simulink model "Demo_veDYNA_cs"  (Simulink 7.6)
settings: Solver=ode1  SolverMode=SingleTasking  StartTime=0  StopTime=15  FixedStep=1/500  RelTol=1e-3
PreLoadFcn:
  | PreScanveDYNAPreLoadFcn(bdroot);
  | check_NUTS_defined;
  | 
  | assignin('base',['model_closed_' bdroot],false);
PostLoadFcn:
  | PreScanveDYNAPostLoadFcn(bdroot);
  | 
InitFcn:
  | vdy_SetExternalInputSource('ManLongCtrl',1,'Brake','other');
  | vdy_SetExternalInputSource('ManLongCtrl',1,'EngineTorque','other');
  | vdy_SetExternalInputSource('ManLatCtrl',1,'Steering','other');
  | 
  | PreScanveDYNAInitFcn(bdroot);
  | PreScanExperimentInitFcn(bdroot)
StopFcn:
  | PreScanExperimentStopFcn(bdroot)
undefined symbols (not defined in the file): at_period, CPT, DiscIntNeverNeededParam, vm_at_pulsewidth, vm_driver_dflt_gain, x_ini_VRML, y_ini_VRML, z_ini_VRML
libraries: dyna_cpt_lib x93, PreScanSimulinkLibrary x10, PreScanUsefulBlocks x4, simulink x4, anilib x3, dyna_lib x3, simulink_extras x2, dyna_manctrl_lib x2, dyna_road_lib x2, dyna_io_lib x1, dyna_demo_lib x1, dyna_usr_maneuver_states_lib x1
(part 6 of 8)

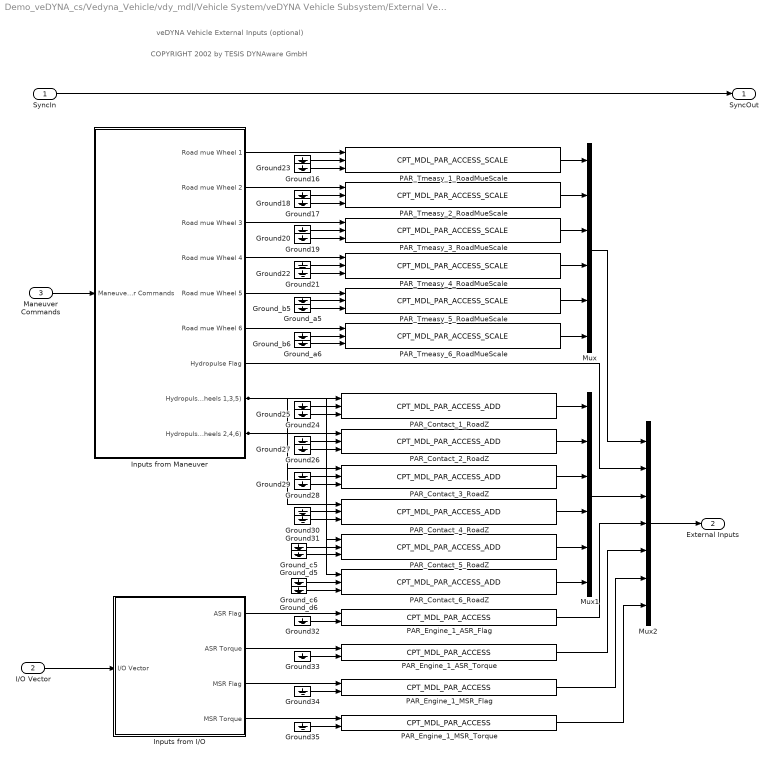
== system Demo_veDYNA_cs/Vedyna_Vehicle/vdy_mdl/Vehicle System/veDYNA Vehicle Subsystem/External Vehicle Inputs (from I/O) ==
  note: COPYRIGHT 2002 by TESIS DYNAware GmbH
  note: veDYNA Vehicle External Inputs (optional)
  SyncIn : Inport
  I/O Vector : Inport  Port=2
  Maneuver Commands : Inport  Port=3
  Ground{16..35} (20 alike) : Ground
  Ground_a5 : Ground
  Ground_a6 : Ground
  Ground_b5 : Ground
  Ground_b6 : Ground
  Ground_c5 : Ground
  Ground_c6 : Ground
  Ground_d5 : Ground
  Ground_d6 : Ground
  Inputs from I/O : Subsystem
  Inputs from Maneuver : Subsystem
  Mux : Mux  Inputs=6
  Mux1 : Mux  Inputs=6
  Mux2 : Mux  Inputs=7
  PAR_Contact_1_RoadZ : dyna_cpt_lib/CPT_MDL_PAR_ACCESS_ADD  Tag=vedynaCPT_MDL_PAR_ACCESS  component=Contact  system_inst=1  parameter=RoadZ
  PAR_Contact_2_RoadZ : dyna_cpt_lib/CPT_MDL_PAR_ACCESS_ADD  Tag=vedynaCPT_MDL_PAR_ACCESS  component=Contact  system_inst=2  parameter=RoadZ
  PAR_Contact_3_RoadZ : dyna_cpt_lib/CPT_MDL_PAR_ACCESS_ADD  Tag=vedynaCPT_MDL_PAR_ACCESS  component=Contact  system_inst=3  parameter=RoadZ
  PAR_Contact_4_RoadZ : dyna_cpt_lib/CPT_MDL_PAR_ACCESS_ADD  Tag=vedynaCPT_MDL_PAR_ACCESS  component=Contact  system_inst=4  parameter=RoadZ
  PAR_Contact_5_RoadZ : dyna_cpt_lib/CPT_MDL_PAR_ACCESS_ADD  Tag=vedynaCPT_MDL_PAR_ACCESS  component=Contact  system_inst=5  parameter=RoadZ
  PAR_Contact_6_RoadZ : dyna_cpt_lib/CPT_MDL_PAR_ACCESS_ADD  Tag=vedynaCPT_MDL_PAR_ACCESS  component=Contact  system_inst=6  parameter=RoadZ
  PAR_Engine_1_ASR_Flag : dyna_cpt_lib/CPT_MDL_PAR_ACCESS  Tag=vedynaCPT_MDL_PAR_ACCESS  component=Engine  system_inst=1  parameter=ASR_Flag
  PAR_Engine_1_ASR_Torque : dyna_cpt_lib/CPT_MDL_PAR_ACCESS  Tag=vedynaCPT_MDL_PAR_ACCESS  component=Engine  system_inst=1  parameter=ASR_Torque
  PAR_Engine_1_MSR_Flag : dyna_cpt_lib/CPT_MDL_PAR_ACCESS  Tag=vedynaCPT_MDL_PAR_ACCESS  component=Engine  system_inst=1  parameter=MSR_Flag
  PAR_Engine_1_MSR_Torque : dyna_cpt_lib/CPT_MDL_PAR_ACCESS  Tag=vedynaCPT_MDL_PAR_ACCESS  component=Engine  system_inst=1  parameter=MSR_Torque
  PAR_Tmeasy_1_RoadMueScale : dyna_cpt_lib/CPT_MDL_PAR_ACCESS_SCALE  Tag=vedynaCPT_MDL_PAR_ACCESS  component=Tmeasy  system_inst=1  parameter=RoadMueScale
  PAR_Tmeasy_2_RoadMueScale : dyna_cpt_lib/CPT_MDL_PAR_ACCESS_SCALE  Tag=vedynaCPT_MDL_PAR_ACCESS  component=Tmeasy  system_inst=2  parameter=RoadMueScale
  PAR_Tmeasy_3_RoadMueScale : dyna_cpt_lib/CPT_MDL_PAR_ACCESS_SCALE  Tag=vedynaCPT_MDL_PAR_ACCESS  component=Tmeasy  system_inst=3  parameter=RoadMueScale
  PAR_Tmeasy_4_RoadMueScale : dyna_cpt_lib/CPT_MDL_PAR_ACCESS_SCALE  Tag=vedynaCPT_MDL_PAR_ACCESS  component=Tmeasy  system_inst=4  parameter=RoadMueScale
  PAR_Tmeasy_5_RoadMueScale : dyna_cpt_lib/CPT_MDL_PAR_ACCESS_SCALE  Tag=vedynaCPT_MDL_PAR_ACCESS  component=Tmeasy  system_inst=5  parameter=RoadMueScale
  PAR_Tmeasy_6_RoadMueScale : dyna_cpt_lib/CPT_MDL_PAR_ACCESS_SCALE  Tag=vedynaCPT_MDL_PAR_ACCESS  component=Tmeasy  system_inst=6  parameter=RoadMueScale
  SyncOut : Outport
  External Inputs : Outport  Port=2
  wires:
  PAR_Contact_6_RoadZ/1 -> Mux1/6
  Ground_d6/1 -> PAR_Contact_6_RoadZ/3
  Ground_c6/1 -> PAR_Contact_6_RoadZ/2
  PAR_Contact_5_RoadZ/1 -> Mux1/5
  Ground_d5/1 -> PAR_Contact_5_RoadZ/3
  Ground_c5/1 -> PAR_Contact_5_RoadZ/2
  Inputs from Maneuver/9(Hydropulse Right (Wheels 2,4,6)) -> PAR_Contact_6_RoadZ/1, PAR_Contact_4_RoadZ/1, PAR_Contact_2_RoadZ/1
  Inputs from Maneuver/8(Hydropulse Left (Wheels 1,3,5)) -> PAR_Contact_5_RoadZ/1, PAR_Contact_3_RoadZ/1, PAR_Contact_1_RoadZ/1
  PAR_Tmeasy_6_RoadMueScale/1 -> Mux/6
  Inputs from Maneuver/6(Road mue Wheel 6) -> PAR_Tmeasy_6_RoadMueScale/1
  Ground_b6/1 -> PAR_Tmeasy_6_RoadMueScale/3
  Ground_a6/1 -> PAR_Tmeasy_6_RoadMueScale/2
  PAR_Tmeasy_5_RoadMueScale/1 -> Mux/5
  Inputs from Maneuver/5(Road mue Wheel 5) -> PAR_Tmeasy_5_RoadMueScale/1
  Ground_b5/1 -> PAR_Tmeasy_5_RoadMueScale/3
  Ground_a5/1 -> PAR_Tmeasy_5_RoadMueScale/2
  Ground16/1 -> PAR_Tmeasy_1_RoadMueScale/2
  Ground17/1 -> PAR_Tmeasy_2_RoadMueScale/2
  Ground18/1 -> PAR_Tmeasy_2_RoadMueScale/3
  Ground19/1 -> PAR_Tmeasy_3_RoadMueScale/2
  Ground20/1 -> PAR_Tmeasy_3_RoadMueScale/3
  Ground21/1 -> PAR_Tmeasy_4_RoadMueScale/2
  Ground22/1 -> PAR_Tmeasy_4_RoadMueScale/3
  Ground23/1 -> PAR_Tmeasy_1_RoadMueScale/3
  Ground24/1 -> PAR_Contact_1_RoadZ/2
  Ground25/1 -> PAR_Contact_1_RoadZ/3
  Ground26/1 -> PAR_Contact_2_RoadZ/2
  Ground27/1 -> PAR_Contact_2_RoadZ/3
  Ground28/1 -> PAR_Contact_3_RoadZ/2
  Ground29/1 -> PAR_Contact_3_RoadZ/3
  Ground30/1 -> PAR_Contact_4_RoadZ/2
  Ground31/1 -> PAR_Contact_4_RoadZ/3
  PAR_Tmeasy_1_RoadMueScale/1 -> Mux/1
  PAR_Tmeasy_2_RoadMueScale/1 -> Mux/2
  PAR_Contact_1_RoadZ/1 -> Mux1/1
  PAR_Contact_2_RoadZ/1 -> Mux1/2
  Inputs from Maneuver/1(Road mue Wheel 1) -> PAR_Tmeasy_1_RoadMueScale/1
  Inputs from Maneuver/2(Road mue Wheel 2) -> PAR_Tmeasy_2_RoadMueScale/1
  Inputs from Maneuver/3(Road mue Wheel 3) -> PAR_Tmeasy_3_RoadMueScale/1
  Inputs from Maneuver/4(Road mue Wheel 4) -> PAR_Tmeasy_4_RoadMueScale/1
  Maneuver Commands/1 -> Inputs from Maneuver/1(Maneuver Commands)
  SyncIn/1 -> SyncOut/1
  Ground32/1 -> PAR_Engine_1_ASR_Flag/2
  Ground33/1 -> PAR_Engine_1_ASR_Torque/2
  Ground34/1 -> PAR_Engine_1_MSR_Flag/2
  Ground35/1 -> PAR_Engine_1_MSR_Torque/2
  I/O Vector/1 -> Inputs from I/O/1(I/O Vector)
  Inputs from I/O/1(ASR Flag) -> PAR_Engine_1_ASR_Flag/1
  Inputs from I/O/2(ASR Torque) -> PAR_Engine_1_ASR_Torque/1
  Inputs from I/O/3(MSR Flag) -> PAR_Engine_1_MSR_Flag/1
  Inputs from I/O/4(MSR Torque) -> PAR_Engine_1_MSR_Torque/1
  PAR_Tmeasy_3_RoadMueScale/1 -> Mux/3
  PAR_Tmeasy_4_RoadMueScale/1 -> Mux/4
  PAR_Contact_3_RoadZ/1 -> Mux1/3
  PAR_Contact_4_RoadZ/1 -> Mux1/4
  Mux/1 -> Mux2/1
  Mux2/1 -> External Inputs/1
  Inputs from Maneuver/7(Hydropulse Flag) -> Mux2/2
  Mux1/1 -> Mux2/3
  PAR_Engine_1_ASR_Flag/1 -> Mux2/4
  PAR_Engine_1_ASR_Torque/1 -> Mux2/5
  PAR_Engine_1_MSR_Flag/1 -> Mux2/6
  PAR_Engine_1_MSR_Torque/1 -> Mux2/7

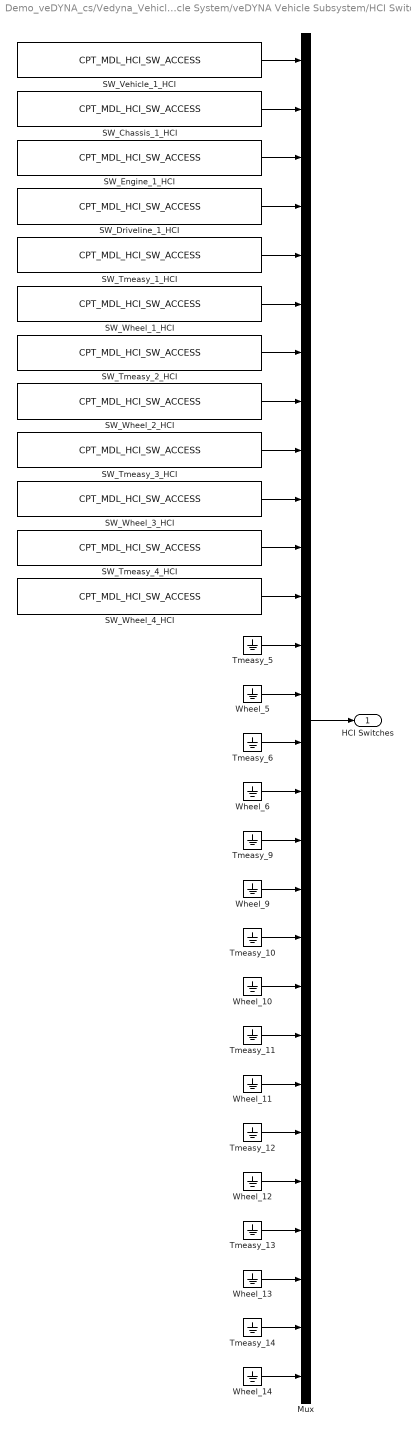
== system Demo_veDYNA_cs/Vedyna_Vehicle/vdy_mdl/Vehicle System/veDYNA Vehicle Subsystem/HCI Switches ==
  Mux : Mux  Inputs=28
  SW_Chassis_1_HCI : dyna_cpt_lib/CPT_MDL_HCI_SW_ACCESS  Tag=vedynaCPT_MDL_HCI_SW_ACCESS  component=Chassis  system_inst=1  parameter=HCI
  SW_Driveline_1_HCI : dyna_cpt_lib/CPT_MDL_HCI_SW_ACCESS  Tag=vedynaCPT_MDL_HCI_SW_ACCESS  component=Driveline  system_inst=1  parameter=HCI
  SW_Engine_1_HCI : dyna_cpt_lib/CPT_MDL_HCI_SW_ACCESS  Tag=vedynaCPT_MDL_HCI_SW_ACCESS  component=Engine  system_inst=1  parameter=HCI
  SW_Tmeasy_1_HCI : dyna_cpt_lib/CPT_MDL_HCI_SW_ACCESS  Tag=vedynaCPT_MDL_HCI_SW_ACCESS  component=Tmeasy  system_inst=1  parameter=HCI
  SW_Tmeasy_2_HCI : dyna_cpt_lib/CPT_MDL_HCI_SW_ACCESS  Tag=vedynaCPT_MDL_HCI_SW_ACCESS  component=Tmeasy  system_inst=2  parameter=HCI
  SW_Tmeasy_3_HCI : dyna_cpt_lib/CPT_MDL_HCI_SW_ACCESS  Tag=vedynaCPT_MDL_HCI_SW_ACCESS  component=Tmeasy  system_inst=3  parameter=HCI
  SW_Tmeasy_4_HCI : dyna_cpt_lib/CPT_MDL_HCI_SW_ACCESS  Tag=vedynaCPT_MDL_HCI_SW_ACCESS  component=Tmeasy  system_inst=4  parameter=HCI
  SW_Vehicle_1_HCI : dyna_cpt_lib/CPT_MDL_HCI_SW_ACCESS  Tag=vedynaCPT_MDL_HCI_SW_ACCESS  component=Vehicle  system_inst=1  parameter=HCI
  SW_Wheel_1_HCI : dyna_cpt_lib/CPT_MDL_HCI_SW_ACCESS  Tag=vedynaCPT_MDL_HCI_SW_ACCESS  component=Wheel  system_inst=1  parameter=HCI
  SW_Wheel_2_HCI : dyna_cpt_lib/CPT_MDL_HCI_SW_ACCESS  Tag=vedynaCPT_MDL_HCI_SW_ACCESS  component=Wheel  system_inst=2  parameter=HCI
  SW_Wheel_3_HCI : dyna_cpt_lib/CPT_MDL_HCI_SW_ACCESS  Tag=vedynaCPT_MDL_HCI_SW_ACCESS  component=Wheel  system_inst=3  parameter=HCI
  SW_Wheel_4_HCI : dyna_cpt_lib/CPT_MDL_HCI_SW_ACCESS  Tag=vedynaCPT_MDL_HCI_SW_ACCESS  component=Wheel  system_inst=4  parameter=HCI
  Tmeasy_{5..6,9..14} (8 alike) : Ground
  Wheel_{5..6,9..14} (8 alike) : Ground
  HCI Switches : Outport
  wires:
  Tmeasy_14/1 -> Mux/27
  Tmeasy_13/1 -> Mux/25
  Wheel_14/1 -> Mux/28
  Wheel_13/1 -> Mux/26
  Wheel_12/1 -> Mux/24
  Tmeasy_12/1 -> Mux/23
  Wheel_11/1 -> Mux/22
  Tmeasy_11/1 -> Mux/21
  Wheel_10/1 -> Mux/20
  Tmeasy_10/1 -> Mux/19
  Wheel_9/1 -> Mux/18
  Tmeasy_9/1 -> Mux/17
  Wheel_6/1 -> Mux/16
  Tmeasy_6/1 -> Mux/15
  Wheel_5/1 -> Mux/14
  Tmeasy_5/1 -> Mux/13
  SW_Wheel_4_HCI/1 -> Mux/12
  SW_Tmeasy_4_HCI/1 -> Mux/11
  SW_Wheel_3_HCI/1 -> Mux/10
  SW_Tmeasy_3_HCI/1 -> Mux/9
  SW_Wheel_2_HCI/1 -> Mux/8
  SW_Tmeasy_2_HCI/1 -> Mux/7
  SW_Wheel_1_HCI/1 -> Mux/6
  SW_Tmeasy_1_HCI/1 -> Mux/5
  SW_Driveline_1_HCI/1 -> Mux/4
  SW_Engine_1_HCI/1 -> Mux/3
  SW_Chassis_1_HCI/1 -> Mux/2
  SW_Vehicle_1_HCI/1 -> Mux/1
  Mux/1 -> HCI Switches/1

== system Demo_veDYNA_cs/Vedyna_Vehicle/vdy_mdl/Vehicle System/veDYNA Vehicle Subsystem/Maneuver Commands Splitter ==
  note: veDYNA Maneuver Command Splitter
  note: COPYRIGHT 2002 by TESIS DYNAware GmbH
  SyncIn : Inport
  Maneuver Commands : Inport  Port=2
  Demux : Demux  Outputs=[1,8,9]
  SyncOut : Outport
  Maneuver Commands to External Inputs : Outport  Port=2
  Maneuver Commands to Brake System : Outport  Port=3
  Maneuver Commands to Vehicle : Outport  Port=4
  wires:
  SyncIn/1 -> SyncOut/1
  Maneuver Commands/1 -> Demux/1
  Demux/3 -> Maneuver Commands to External Inputs/1
  Demux/1 -> Maneuver Commands to Brake System/1
  Demux/2 -> Maneuver Commands to Vehicle/1

== system Demo_veDYNA_cs/Vedyna_Vehicle/vdy_mdl/Vehicle System/veDYNA Vehicle Subsystem/Vehicle Outputs to I/O ==
  note: COPYRIGHT 2002 by TESIS DYNAware GmbH
  note: veDYNA Vehicle Interface to I/O (optional)
  SyncIn : Inport
  Read From WorkSpace : dyna_lib/Read From WorkSpace  comp=Wheel|Wheel|Wheel|Wheel|Wheel|Wheel|Wheel|Wheel  inst=0|1|2|3|4|5|6|7  group=wheelstate_v|wheelstate_v|wheelstate_v|wheelstate_v|wheelstate_v|wheelstate_v|wheelstate_v|wheelstate_v  var=or|or|or|or|or|or|or|or
  Output to IO : Outport
  SyncOut : Outport  Port=2
  wires:
  SyncIn/1 -> SyncOut/1
  Read From WorkSpace/1 -> Output to IO/1

== system Demo_veDYNA_cs/BMW_X5_1/Trajectories/Traj2State1/Traj2State2/Traj2MuxState_Ext/demux ==
  traj : Inport
  Demux : Demux  Outputs=18
  x : Outport
  y : Outport  Port=2
  z : Outport  Port=3
  velx : Outport  Port=4
  vely : Outport  Port=5
  velz : Outport  Port=6
  R : Outport  Port=7
  P : Outport  Port=8
  Y : Outport  Port=9
  velR : Outport  Port=10
  velP : Outport  Port=11
  velY : Outport  Port=12
  accx : Outport  Port=13
  accy : Outport  Port=14
  accz : Outport  Port=15
  accR : Outport  Port=16
  accP : Outport  Port=17
  accY : Outport  Port=18
  wires:
  Demux/18 -> accY/1
  Demux/17 -> accP/1
  Demux/16 -> accR/1
  Demux/15 -> accz/1
  Demux/14 -> accy/1
  Demux/13 -> accx/1
  Demux/12 -> velY/1
  Demux/11 -> velP/1
  Demux/10 -> velR/1
  Demux/9 -> velz/1
  Demux/8 -> vely/1
  Demux/7 -> velx/1
  Demux/6 -> Y/1
  Demux/5 -> P/1
  traj/1 -> Demux/1
  Demux/4 -> R/1
  Demux/3 -> z/1
  Demux/2 -> y/1
  Demux/1 -> x/1

== system Demo_veDYNA_cs/Nissan_Cabstar_1/Trajectories/Traj2State1/Traj2State2/Traj2MuxState_Ext/demux ==
  traj : Inport
  Demux : Demux  Outputs=18
  x : Outport
  y : Outport  Port=2
  z : Outport  Port=3
  velx : Outport  Port=4
  vely : Outport  Port=5
  velz : Outport  Port=6
  R : Outport  Port=7
  P : Outport  Port=8
  Y : Outport  Port=9
  velR : Outport  Port=10
  velP : Outport  Port=11
  velY : Outport  Port=12
  accx : Outport  Port=13
  accy : Outport  Port=14
  accz : Outport  Port=15
  accR : Outport  Port=16
  accP : Outport  Port=17
  accY : Outport  Port=18
  wires:
  Demux/18 -> accY/1
  Demux/17 -> accP/1
  Demux/16 -> accR/1
  Demux/15 -> accz/1
  Demux/14 -> accy/1
  Demux/13 -> accx/1
  Demux/12 -> velY/1
  Demux/11 -> velP/1
  Demux/10 -> velR/1
  Demux/9 -> velz/1
  Demux/8 -> vely/1
  Demux/7 -> velx/1
  Demux/6 -> Y/1
  Demux/5 -> P/1
  traj/1 -> Demux/1
  Demux/4 -> R/1
  Demux/3 -> z/1
  Demux/2 -> y/1
  Demux/1 -> x/1

== system Demo_veDYNA_cs/Vedyna_Vehicle/CPT_MDL/MDL_PAR/BrkHyd/System Instance 1/pbrmaster [N/m**2] ==
  Table : Lookup  InputValues=CPT.MDL_PAR.BrkHyd{1}.pbrmaster.Table.x  Table=CPT.MDL_PAR.BrkHyd{1}.pbrmaster.Table.v  SaturateOnIntegerOverflow=on
  Terminator : Terminator
  Terminator1 : Terminator
  Value : Constant  Value=CPT.MDL_PAR.BrkHyd{1}.pbrmaster.Value.v
  tag scope: BrkHyd_1_pbrmaster_TBL=global, BrkHyd_1_pbrmaster_VAL=global
  wires:
  [vdy_Simctrl_tsim] -> Table/1
  Value/1 -> [BrkHyd_1_pbrmaster_VAL]
  [BrkHyd_1_pbrmaster_VAL] -> Terminator/1
  [BrkHyd_1_pbrmaster_TBL] -> Terminator1/1
  Table/1 -> [BrkHyd_1_pbrmaster_TBL]

== system Demo_veDYNA_cs/Vedyna_Vehicle/CPT_MDL/MDL_PAR/ClutchCtrl/System Instance 1/Clutch [%] ==
  Table : Lookup  InputValues=CPT.MDL_PAR.ClutchCtrl{1}.Clutch.Table.x  Table=CPT.MDL_PAR.ClutchCtrl{1}.Clutch.Table.v  SaturateOnIntegerOverflow=on
  Terminator : Terminator
  Terminator1 : Terminator
  Value : Constant  Value=CPT.MDL_PAR.ClutchCtrl{1}.Clutch.Value.v
  tag scope: ClutchCtrl_1_Clutch_TBL=global, ClutchCtrl_1_Clutch_VAL=global
  wires:
  [vdy_Simctrl_tsim] -> Table/1
  Value/1 -> [ClutchCtrl_1_Clutch_VAL]
  [ClutchCtrl_1_Clutch_VAL] -> Terminator/1
  [ClutchCtrl_1_Clutch_TBL] -> Terminator1/1
  Table/1 -> [ClutchCtrl_1_Clutch_TBL]

== system Demo_veDYNA_cs/Vedyna_Vehicle/CPT_MDL/MDL_PAR/Contact/System Instance 1/RoadZ [m] ==
  Table : Lookup  InputValues=CPT.MDL_PAR.Contact{1}.RoadZ.Table.x  Table=CPT.MDL_PAR.Contact{1}.RoadZ.Table.v  SaturateOnIntegerOverflow=on
  Terminator : Terminator
  Terminator1 : Terminator
  Value : Constant  Value=CPT.MDL_PAR.Contact{1}.RoadZ.Value.v
  tag scope: Contact_1_RoadZ_TBL=global, Contact_1_RoadZ_VAL=global
  wires:
  [vdy_Simctrl_tsim] -> Table/1
  Value/1 -> [Contact_1_RoadZ_VAL]
  [Contact_1_RoadZ_VAL] -> Terminator/1
  [Contact_1_RoadZ_TBL] -> Terminator1/1
  Table/1 -> [Contact_1_RoadZ_TBL]

== system Demo_veDYNA_cs/Vedyna_Vehicle/CPT_MDL/MDL_PAR/Contact/System Instance 2/RoadZ [m] ==
  Table : Lookup  InputValues=CPT.MDL_PAR.Contact{2}.RoadZ.Table.x  Table=CPT.MDL_PAR.Contact{2}.RoadZ.Table.v  SaturateOnIntegerOverflow=on
  Terminator : Terminator
  Terminator1 : Terminator
  Value : Constant  Value=CPT.MDL_PAR.Contact{2}.RoadZ.Value.v
  tag scope: Contact_2_RoadZ_TBL=global, Contact_2_RoadZ_VAL=global
  wires:
  [vdy_Simctrl_tsim] -> Table/1
  Value/1 -> [Contact_2_RoadZ_VAL]
  [Contact_2_RoadZ_VAL] -> Terminator/1
  [Contact_2_RoadZ_TBL] -> Terminator1/1
  Table/1 -> [Contact_2_RoadZ_TBL]

== system Demo_veDYNA_cs/Vedyna_Vehicle/CPT_MDL/MDL_PAR/Contact/System Instance 3/RoadZ [m] ==
  Table : Lookup  InputValues=CPT.MDL_PAR.Contact{3}.RoadZ.Table.x  Table=CPT.MDL_PAR.Contact{3}.RoadZ.Table.v  SaturateOnIntegerOverflow=on
  Terminator : Terminator
  Terminator1 : Terminator
  Value : Constant  Value=CPT.MDL_PAR.Contact{3}.RoadZ.Value.v
  tag scope: Contact_3_RoadZ_TBL=global, Contact_3_RoadZ_VAL=global
  wires:
  [vdy_Simctrl_tsim] -> Table/1
  Value/1 -> [Contact_3_RoadZ_VAL]
  [Contact_3_RoadZ_VAL] -> Terminator/1
  [Contact_3_RoadZ_TBL] -> Terminator1/1
  Table/1 -> [Contact_3_RoadZ_TBL]

== system Demo_veDYNA_cs/Vedyna_Vehicle/CPT_MDL/MDL_PAR/Contact/System Instance 4/RoadZ [m] ==
  Table : Lookup  InputValues=CPT.MDL_PAR.Contact{4}.RoadZ.Table.x  Table=CPT.MDL_PAR.Contact{4}.RoadZ.Table.v  SaturateOnIntegerOverflow=on
  Terminator : Terminator
  Terminator1 : Terminator
  Value : Constant  Value=CPT.MDL_PAR.Contact{4}.RoadZ.Value.v
  tag scope: Contact_4_RoadZ_TBL=global, Contact_4_RoadZ_VAL=global
  wires:
  [vdy_Simctrl_tsim] -> Table/1
  Value/1 -> [Contact_4_RoadZ_VAL]
  [Contact_4_RoadZ_VAL] -> Terminator/1
  [Contact_4_RoadZ_TBL] -> Terminator1/1
  Table/1 -> [Contact_4_RoadZ_TBL]

== system Demo_veDYNA_cs/Vedyna_Vehicle/CPT_MDL/MDL_PAR/Contact/System Instance 5/RoadZ [m] ==
  Table : Lookup  InputValues=CPT.MDL_PAR.Contact{5}.RoadZ.Table.x  Table=CPT.MDL_PAR.Contact{5}.RoadZ.Table.v  SaturateOnIntegerOverflow=on
  Terminator : Terminator
  Terminator1 : Terminator
  Value : Constant  Value=CPT.MDL_PAR.Contact{5}.RoadZ.Value.v
  tag scope: Contact_5_RoadZ_TBL=global, Contact_5_RoadZ_VAL=global
  wires:
  [vdy_Simctrl_tsim] -> Table/1
  Value/1 -> [Contact_5_RoadZ_VAL]
  [Contact_5_RoadZ_VAL] -> Terminator/1
  [Contact_5_RoadZ_TBL] -> Terminator1/1
  Table/1 -> [Contact_5_RoadZ_TBL]

== system Demo_veDYNA_cs/Vedyna_Vehicle/CPT_MDL/MDL_PAR/Contact/System Instance 6/RoadZ [m] ==
  Table : Lookup  InputValues=CPT.MDL_PAR.Contact{6}.RoadZ.Table.x  Table=CPT.MDL_PAR.Contact{6}.RoadZ.Table.v  SaturateOnIntegerOverflow=on
  Terminator : Terminator
  Terminator1 : Terminator
  Value : Constant  Value=CPT.MDL_PAR.Contact{6}.RoadZ.Value.v
  tag scope: Contact_6_RoadZ_TBL=global, Contact_6_RoadZ_VAL=global
  wires:
  [vdy_Simctrl_tsim] -> Table/1
  Value/1 -> [Contact_6_RoadZ_VAL]
  [Contact_6_RoadZ_VAL] -> Terminator/1
  [Contact_6_RoadZ_TBL] -> Terminator1/1
  Table/1 -> [Contact_6_RoadZ_TBL]

== system Demo_veDYNA_cs/Vedyna_Vehicle/CPT_MDL/MDL_PAR/Contact/System Instance 7/RoadZ [m] ==
  Table : Lookup  InputValues=CPT.MDL_PAR.Contact{7}.RoadZ.Table.x  Table=CPT.MDL_PAR.Contact{7}.RoadZ.Table.v  SaturateOnIntegerOverflow=on
  Terminator : Terminator
  Terminator1 : Terminator
  Value : Constant  Value=CPT.MDL_PAR.Contact{7}.RoadZ.Value.v
  tag scope: Contact_7_RoadZ_TBL=global, Contact_7_RoadZ_VAL=global
  wires:
  [vdy_Simctrl_tsim] -> Table/1
  Value/1 -> [Contact_7_RoadZ_VAL]
  [Contact_7_RoadZ_VAL] -> Terminator/1
  [Contact_7_RoadZ_TBL] -> Terminator1/1
  Table/1 -> [Contact_7_RoadZ_TBL]

== system Demo_veDYNA_cs/Vedyna_Vehicle/CPT_MDL/MDL_PAR/Contact/System Instance 8/RoadZ [m] ==
  Table : Lookup  InputValues=CPT.MDL_PAR.Contact{8}.RoadZ.Table.x  Table=CPT.MDL_PAR.Contact{8}.RoadZ.Table.v  SaturateOnIntegerOverflow=on
  Terminator : Terminator
  Terminator1 : Terminator
  Value : Constant  Value=CPT.MDL_PAR.Contact{8}.RoadZ.Value.v
  tag scope: Contact_8_RoadZ_TBL=global, Contact_8_RoadZ_VAL=global
  wires:
  [vdy_Simctrl_tsim] -> Table/1
  Value/1 -> [Contact_8_RoadZ_VAL]
  [Contact_8_RoadZ_VAL] -> Terminator/1
  [Contact_8_RoadZ_TBL] -> Terminator1/1
  Table/1 -> [Contact_8_RoadZ_TBL]

== system Demo_veDYNA_cs/Vedyna_Vehicle/CPT_MDL/MDL_PAR/Driver/System Instance 1/acc_comp_scale [-] ==
  Table : Lookup  InputValues=CPT.MDL_PAR.Driver{1}.acc_comp_scale.Table.x  Table=CPT.MDL_PAR.Driver{1}.acc_comp_scale.Table.v  SaturateOnIntegerOverflow=on
  Terminator : Terminator
  Terminator1 : Terminator
  Value : Constant  Value=CPT.MDL_PAR.Driver{1}.acc_comp_scale.Value.v
  tag scope: Driver_1_acc_comp_scale_TBL=global, Driver_1_acc_comp_scale_VAL=global
  wires:
  [vdy_Simctrl_tsim] -> Table/1
  Value/1 -> [Driver_1_acc_comp_scale_VAL]
  [Driver_1_acc_comp_scale_VAL] -> Terminator/1
  [Driver_1_acc_comp_scale_TBL] -> Terminator1/1
  Table/1 -> [Driver_1_acc_comp_scale_TBL]

== system Demo_veDYNA_cs/Vedyna_Vehicle/CPT_MDL/MDL_PAR/Driver/System Instance 1/adj_acc_gain [-] ==
  Table : Lookup  InputValues=CPT.MDL_PAR.Driver{1}.adj_acc_gain.Table.x  Table=CPT.MDL_PAR.Driver{1}.adj_acc_gain.Table.v  SaturateOnIntegerOverflow=on
  Terminator : Terminator
  Terminator1 : Terminator
  Value : Constant  Value=CPT.MDL_PAR.Driver{1}.adj_acc_gain.Value.v
  tag scope: Driver_1_adj_acc_gain_TBL=global, Driver_1_adj_acc_gain_VAL=global
  wires:
  [vdy_Simctrl_tsim] -> Table/1
  Value/1 -> [Driver_1_adj_acc_gain_VAL]
  [Driver_1_adj_acc_gain_VAL] -> Terminator/1
  [Driver_1_adj_acc_gain_TBL] -> Terminator1/1
  Table/1 -> [Driver_1_adj_acc_gain_TBL]

== system Demo_veDYNA_cs/Vedyna_Vehicle/CPT_MDL/MDL_PAR/Driver/System Instance 1/adj_brake_gain [-] ==
  Table : Lookup  InputValues=CPT.MDL_PAR.Driver{1}.adj_brake_gain.Table.x  Table=CPT.MDL_PAR.Driver{1}.adj_brake_gain.Table.v  SaturateOnIntegerOverflow=on
  Terminator : Terminator
  Terminator1 : Terminator
  Value : Constant  Value=CPT.MDL_PAR.Driver{1}.adj_brake_gain.Value.v
  tag scope: Driver_1_adj_brake_gain_TBL=global, Driver_1_adj_brake_gain_VAL=global
  wires:
  [vdy_Simctrl_tsim] -> Table/1
  Value/1 -> [Driver_1_adj_brake_gain_VAL]
  [Driver_1_adj_brake_gain_VAL] -> Terminator/1
  [Driver_1_adj_brake_gain_TBL] -> Terminator1/1
  Table/1 -> [Driver_1_adj_brake_gain_TBL]

== system Demo_veDYNA_cs/Vedyna_Vehicle/CPT_MDL/MDL_PAR/Driver/System Instance 1/ax_min [m/s^2] ==
  Table : Lookup  InputValues=CPT.MDL_PAR.Driver{1}.ax_min.Table.x  Table=CPT.MDL_PAR.Driver{1}.ax_min.Table.v  SaturateOnIntegerOverflow=on
  Terminator : Terminator
  Terminator1 : Terminator
  Value : Constant  Value=CPT.MDL_PAR.Driver{1}.ax_min.Value.v
  tag scope: Driver_1_ax_min_TBL=global, Driver_1_ax_min_VAL=global
  wires:
  [vdy_Simctrl_tsim] -> Table/1
  Value/1 -> [Driver_1_ax_min_VAL]
  [Driver_1_ax_min_VAL] -> Terminator/1
  [Driver_1_ax_min_TBL] -> Terminator1/1
  Table/1 -> [Driver_1_ax_min_TBL]

== system Demo_veDYNA_cs/Vedyna_Vehicle/CPT_MDL/MDL_PAR/Driver/System Instance 1/ctrl_acc_smooth_t [s] ==
  Table : Lookup  InputValues=CPT.MDL_PAR.Driver{1}.ctrl_acc_smooth_t.Table.x  Table=CPT.MDL_PAR.Driver{1}.ctrl_acc_smooth_t.Table.v  SaturateOnIntegerOverflow=on
  Terminator : Terminator
  Terminator1 : Terminator
  Value : Constant  Value=CPT.MDL_PAR.Driver{1}.ctrl_acc_smooth_t.Value.v
  tag scope: Driver_1_ctrl_acc_smooth_t_TBL=global, Driver_1_ctrl_acc_smooth_t_VAL=global
  wires:
  [vdy_Simctrl_tsim] -> Table/1
  Value/1 -> [Driver_1_ctrl_acc_smooth_t_VAL]
  [Driver_1_ctrl_acc_smooth_t_VAL] -> Terminator/1
  [Driver_1_ctrl_acc_smooth_t_TBL] -> Terminator1/1
  Table/1 -> [Driver_1_ctrl_acc_smooth_t_TBL]

== system Demo_veDYNA_cs/Vedyna_Vehicle/CPT_MDL/MDL_PAR/Driver/System Instance 1/cu_comp_scale [-] ==
  Table : Lookup  InputValues=CPT.MDL_PAR.Driver{1}.cu_comp_scale.Table.x  Table=CPT.MDL_PAR.Driver{1}.cu_comp_scale.Table.v  SaturateOnIntegerOverflow=on
  Terminator : Terminator
  Terminator1 : Terminator
  Value : Constant  Value=CPT.MDL_PAR.Driver{1}.cu_comp_scale.Value.v
  tag scope: Driver_1_cu_comp_scale_TBL=global, Driver_1_cu_comp_scale_VAL=global
  wires:
  [vdy_Simctrl_tsim] -> Table/1
  Value/1 -> [Driver_1_cu_comp_scale_VAL]
  [Driver_1_cu_comp_scale_VAL] -> Terminator/1
  [Driver_1_cu_comp_scale_TBL] -> Terminator1/1
  Table/1 -> [Driver_1_cu_comp_scale_TBL]

== system Demo_veDYNA_cs/Vedyna_Vehicle/CPT_MDL/MDL_PAR/Driver/System Instance 1/cu_path [1/m] ==
  Table : Lookup  InputValues=CPT.MDL_PAR.Driver{1}.cu_path.Table.x  Table=CPT.MDL_PAR.Driver{1}.cu_path.Table.v  SaturateOnIntegerOverflow=on
  Terminator : Terminator
  Terminator1 : Terminator
  Value : Constant  Value=CPT.MDL_PAR.Driver{1}.cu_path.Value.v
  tag scope: Driver_1_cu_path_TBL=global, Driver_1_cu_path_VAL=global
  wires:
  [vdy_Driver_s] -> Table/1
  Value/1 -> [Driver_1_cu_path_VAL]
  [Driver_1_cu_path_VAL] -> Terminator/1
  [Driver_1_cu_path_TBL] -> Terminator1/1
  Table/1 -> [Driver_1_cu_path_TBL]

== system Demo_veDYNA_cs/Vedyna_Vehicle/CPT_MDL/MDL_PAR/Driver/System Instance 1/front_stiff [N/rad] ==
  Table : Lookup  InputValues=CPT.MDL_PAR.Driver{1}.front_stiff.Table.x  Table=CPT.MDL_PAR.Driver{1}.front_stiff.Table.v  SaturateOnIntegerOverflow=on
  Terminator : Terminator
  Terminator1 : Terminator
  Value : Constant  Value=CPT.MDL_PAR.Driver{1}.front_stiff.Value.v
  tag scope: Driver_1_front_stiff_TBL=global, Driver_1_front_stiff_VAL=global
  wires:
  [vdy_Simctrl_tsim] -> Table/1
  Value/1 -> [Driver_1_front_stiff_VAL]
  [Driver_1_front_stiff_VAL] -> Terminator/1
  [Driver_1_front_stiff_TBL] -> Terminator1/1
  Table/1 -> [Driver_1_front_stiff_TBL]

== system Demo_veDYNA_cs/Vedyna_Vehicle/CPT_MDL/MDL_PAR/Driver/System Instance 1/front_stiff_sw [-] ==
  Table : Lookup  InputValues=CPT.MDL_PAR.Driver{1}.front_stiff_sw.Table.x  Table=CPT.MDL_PAR.Driver{1}.front_stiff_sw.Table.v  SaturateOnIntegerOverflow=on
  Terminator : Terminator
  Terminator1 : Terminator
  Value : Constant  Value=CPT.MDL_PAR.Driver{1}.front_stiff_sw.Value.v
  tag scope: Driver_1_front_stiff_sw_TBL=global, Driver_1_front_stiff_sw_VAL=global
  wires:
  [vdy_Simctrl_tsim] -> Table/1
  Value/1 -> [Driver_1_front_stiff_sw_VAL]
  [Driver_1_front_stiff_sw_VAL] -> Terminator/1
  [Driver_1_front_stiff_sw_TBL] -> Terminator1/1
  Table/1 -> [Driver_1_front_stiff_sw_TBL]

== system Demo_veDYNA_cs/Vedyna_Vehicle/CPT_MDL/MDL_PAR/Driver/System Instance 1/gain_lat [-] ==
  Table : Lookup  InputValues=CPT.MDL_PAR.Driver{1}.gain_lat.Table.x  Table=CPT.MDL_PAR.Driver{1}.gain_lat.Table.v  SaturateOnIntegerOverflow=on
  Terminator : Terminator
  Terminator1 : Terminator
  Value : Constant  Value=CPT.MDL_PAR.Driver{1}.gain_lat.Value.v
  tag scope: Driver_1_gain_lat_TBL=global, Driver_1_gain_lat_VAL=global
  wires:
  [vdy_Simctrl_tsim] -> Table/1
  Value/1 -> [Driver_1_gain_lat_VAL]
  [Driver_1_gain_lat_VAL] -> Terminator/1
  [Driver_1_gain_lat_TBL] -> Terminator1/1
  Table/1 -> [Driver_1_gain_lat_TBL]

== system Demo_veDYNA_cs/Vedyna_Vehicle/CPT_MDL/MDL_PAR/Driver/System Instance 1/gain_long [-] ==
  Table : Lookup  InputValues=CPT.MDL_PAR.Driver{1}.gain_long.Table.x  Table=CPT.MDL_PAR.Driver{1}.gain_long.Table.v  SaturateOnIntegerOverflow=on
  Terminator : Terminator
  Terminator1 : Terminator
  Value : Constant  Value=CPT.MDL_PAR.Driver{1}.gain_long.Value.v
  tag scope: Driver_1_gain_long_TBL=global, Driver_1_gain_long_VAL=global
  wires:
  [vdy_Simctrl_tsim] -> Table/1
  Value/1 -> [Driver_1_gain_long_VAL]
  [Driver_1_gain_long_VAL] -> Terminator/1
  [Driver_1_gain_long_TBL] -> Terminator1/1
  Table/1 -> [Driver_1_gain_long_TBL]

== system Demo_veDYNA_cs/Vedyna_Vehicle/CPT_MDL/MDL_PAR/Driver/System Instance 1/lat_for_r_scale [-] ==
  Table : Lookup  InputValues=CPT.MDL_PAR.Driver{1}.lat_for_r_scale.Table.x  Table=CPT.MDL_PAR.Driver{1}.lat_for_r_scale.Table.v  SaturateOnIntegerOverflow=on
  Terminator : Terminator
  Terminator1 : Terminator
  Value : Constant  Value=CPT.MDL_PAR.Driver{1}.lat_for_r_scale.Value.v
  tag scope: Driver_1_lat_for_r_scale_TBL=global, Driver_1_lat_for_r_scale_VAL=global
  wires:
  [vdy_Simctrl_tsim] -> Table/1
  Value/1 -> [Driver_1_lat_for_r_scale_VAL]
  [Driver_1_lat_for_r_scale_VAL] -> Terminator/1
  [Driver_1_lat_for_r_scale_TBL] -> Terminator1/1
  Table/1 -> [Driver_1_lat_for_r_scale_TBL]

== system Demo_veDYNA_cs/Vedyna_Vehicle/CPT_MDL/MDL_PAR/Driver/System Instance 1/lat_for_r_smooth_t [s] ==
  Table : Lookup  InputValues=CPT.MDL_PAR.Driver{1}.lat_for_r_smooth_t.Table.x  Table=CPT.MDL_PAR.Driver{1}.lat_for_r_smooth_t.Table.v  SaturateOnIntegerOverflow=on
  Terminator : Terminator
  Terminator1 : Terminator
  Value : Constant  Value=CPT.MDL_PAR.Driver{1}.lat_for_r_smooth_t.Value.v
  tag scope: Driver_1_lat_for_r_smooth_t_TBL=global, Driver_1_lat_for_r_smooth_t_VAL=global
  wires:
  [vdy_Simctrl_tsim] -> Table/1
  Value/1 -> [Driver_1_lat_for_r_smooth_t_VAL]
  [Driver_1_lat_for_r_smooth_t_VAL] -> Terminator/1
  [Driver_1_lat_for_r_smooth_t_TBL] -> Terminator1/1
  Table/1 -> [Driver_1_lat_for_r_smooth_t_TBL]

== system Demo_veDYNA_cs/Vedyna_Vehicle/CPT_MDL/MDL_PAR/Driver/System Instance 1/lat_for_r_sw [-] ==
  Table : Lookup  InputValues=CPT.MDL_PAR.Driver{1}.lat_for_r_sw.Table.x  Table=CPT.MDL_PAR.Driver{1}.lat_for_r_sw.Table.v  SaturateOnIntegerOverflow=on
  Terminator : Terminator
  Terminator1 : Terminator
  Value : Constant  Value=CPT.MDL_PAR.Driver{1}.lat_for_r_sw.Value.v
  tag scope: Driver_1_lat_for_r_sw_TBL=global, Driver_1_lat_for_r_sw_VAL=global
  wires:
  [vdy_Simctrl_tsim] -> Table/1
  Value/1 -> [Driver_1_lat_for_r_sw_VAL]
  [Driver_1_lat_for_r_sw_VAL] -> Terminator/1
  [Driver_1_lat_for_r_sw_TBL] -> Terminator1/1
  Table/1 -> [Driver_1_lat_for_r_sw_TBL]

== system Demo_veDYNA_cs/Vedyna_Vehicle/CPT_MDL/MDL_PAR/Driver/System Instance 1/path_v_scale [-] ==
  Table : Lookup  InputValues=CPT.MDL_PAR.Driver{1}.path_v_scale.Table.x  Table=CPT.MDL_PAR.Driver{1}.path_v_scale.Table.v  SaturateOnIntegerOverflow=on
  Terminator : Terminator
  Terminator1 : Terminator
  Value : Constant  Value=CPT.MDL_PAR.Driver{1}.path_v_scale.Value.v
  tag scope: Driver_1_path_v_scale_TBL=global, Driver_1_path_v_scale_VAL=global
  wires:
  [vdy_Simctrl_tsim] -> Table/1
  Value/1 -> [Driver_1_path_v_scale_VAL]
  [Driver_1_path_v_scale_VAL] -> Terminator/1
  [Driver_1_path_v_scale_TBL] -> Terminator1/1
  Table/1 -> [Driver_1_path_v_scale_TBL]

== system Demo_veDYNA_cs/Vedyna_Vehicle/CPT_MDL/MDL_PAR/Driver/System Instance 1/path_x_offset [m] ==
  Table : Lookup  InputValues=CPT.MDL_PAR.Driver{1}.path_x_offset.Table.x  Table=CPT.MDL_PAR.Driver{1}.path_x_offset.Table.v  SaturateOnIntegerOverflow=on
  Terminator : Terminator
  Terminator1 : Terminator
  Value : Constant  Value=CPT.MDL_PAR.Driver{1}.path_x_offset.Value.v
  tag scope: Driver_1_path_x_offset_TBL=global, Driver_1_path_x_offset_VAL=global
  wires:
  [vdy_Simctrl_tsim] -> Table/1
  Value/1 -> [Driver_1_path_x_offset_VAL]
  [Driver_1_path_x_offset_VAL] -> Terminator/1
  [Driver_1_path_x_offset_TBL] -> Terminator1/1
  Table/1 -> [Driver_1_path_x_offset_TBL]

== system Demo_veDYNA_cs/Vedyna_Vehicle/CPT_MDL/MDL_PAR/Driver/System Instance 1/psi_path [rad] ==
  Table : Lookup  InputValues=CPT.MDL_PAR.Driver{1}.psi_path.Table.x  Table=CPT.MDL_PAR.Driver{1}.psi_path.Table.v  SaturateOnIntegerOverflow=on
  Terminator : Terminator
  Terminator1 : Terminator
  Value : Constant  Value=CPT.MDL_PAR.Driver{1}.psi_path.Value.v
  tag scope: Driver_1_psi_path_TBL=global, Driver_1_psi_path_VAL=global
  wires:
  [vdy_Driver_s] -> Table/1
  Value/1 -> [Driver_1_psi_path_VAL]
  [Driver_1_psi_path_VAL] -> Terminator/1
  [Driver_1_psi_path_TBL] -> Terminator1/1
  Table/1 -> [Driver_1_psi_path_TBL]

== system Demo_veDYNA_cs/Vedyna_Vehicle/CPT_MDL/MDL_PAR/Driver/System Instance 1/q_path [m] ==
  Table : Lookup  InputValues=CPT.MDL_PAR.Driver{1}.q_path.Table.x  Table=CPT.MDL_PAR.Driver{1}.q_path.Table.v  SaturateOnIntegerOverflow=on
  Terminator : Terminator
  Terminator1 : Terminator
  Value : Constant  Value=CPT.MDL_PAR.Driver{1}.q_path.Value.v
  tag scope: Driver_1_q_path_TBL=global, Driver_1_q_path_VAL=global
  wires:
  [vdy_Driver_s] -> Table/1
  Value/1 -> [Driver_1_q_path_VAL]
  [Driver_1_q_path_VAL] -> Terminator/1
  [Driver_1_q_path_TBL] -> Terminator1/1
  Table/1 -> [Driver_1_q_path_TBL]

== system Demo_veDYNA_cs/Vedyna_Vehicle/CPT_MDL/MDL_PAR/Driver/System Instance 1/rear_stiff [N/rad] ==
  Table : Lookup  InputValues=CPT.MDL_PAR.Driver{1}.rear_stiff.Table.x  Table=CPT.MDL_PAR.Driver{1}.rear_stiff.Table.v  SaturateOnIntegerOverflow=on
  Terminator : Terminator
  Terminator1 : Terminator
  Value : Constant  Value=CPT.MDL_PAR.Driver{1}.rear_stiff.Value.v
  tag scope: Driver_1_rear_stiff_TBL=global, Driver_1_rear_stiff_VAL=global
  wires:
  [vdy_Simctrl_tsim] -> Table/1
  Value/1 -> [Driver_1_rear_stiff_VAL]
  [Driver_1_rear_stiff_VAL] -> Terminator/1
  [Driver_1_rear_stiff_TBL] -> Terminator1/1
  Table/1 -> [Driver_1_rear_stiff_TBL]

== system Demo_veDYNA_cs/Vedyna_Vehicle/CPT_MDL/MDL_PAR/Driver/System Instance 1/rear_stiff_sw [-] ==
  Table : Lookup  InputValues=CPT.MDL_PAR.Driver{1}.rear_stiff_sw.Table.x  Table=CPT.MDL_PAR.Driver{1}.rear_stiff_sw.Table.v  SaturateOnIntegerOverflow=on
  Terminator : Terminator
  Terminator1 : Terminator
  Value : Constant  Value=CPT.MDL_PAR.Driver{1}.rear_stiff_sw.Value.v
  tag scope: Driver_1_rear_stiff_sw_TBL=global, Driver_1_rear_stiff_sw_VAL=global
  wires:
  [vdy_Simctrl_tsim] -> Table/1
  Value/1 -> [Driver_1_rear_stiff_sw_VAL]
  [Driver_1_rear_stiff_sw_VAL] -> Terminator/1
  [Driver_1_rear_stiff_sw_TBL] -> Terminator1/1
  Table/1 -> [Driver_1_rear_stiff_sw_TBL]

== system Demo_veDYNA_cs/Vedyna_Vehicle/CPT_MDL/MDL_PAR/Driver/System Instance 1/steer_max [deg] ==
  Table : Lookup  InputValues=CPT.MDL_PAR.Driver{1}.steer_max.Table.x  Table=CPT.MDL_PAR.Driver{1}.steer_max.Table.v  SaturateOnIntegerOverflow=on
  Terminator : Terminator
  Terminator1 : Terminator
  Value : Constant  Value=CPT.MDL_PAR.Driver{1}.steer_max.Value.v
  tag scope: Driver_1_steer_max_TBL=global, Driver_1_steer_max_VAL=global
  wires:
  [vdy_Simctrl_tsim] -> Table/1
  Value/1 -> [Driver_1_steer_max_VAL]
  [Driver_1_steer_max_VAL] -> Terminator/1
  [Driver_1_steer_max_TBL] -> Terminator1/1
  Table/1 -> [Driver_1_steer_max_TBL]

== system Demo_veDYNA_cs/Vedyna_Vehicle/CPT_MDL/MDL_PAR/Driver/System Instance 1/steer_min [deg] ==
  Table : Lookup  InputValues=CPT.MDL_PAR.Driver{1}.steer_min.Table.x  Table=CPT.MDL_PAR.Driver{1}.steer_min.Table.v  SaturateOnIntegerOverflow=on
  Terminator : Terminator
  Terminator1 : Terminator
  Value : Constant  Value=CPT.MDL_PAR.Driver{1}.steer_min.Value.v
  tag scope: Driver_1_steer_min_TBL=global, Driver_1_steer_min_VAL=global
  wires:
  [vdy_Simctrl_tsim] -> Table/1
  Value/1 -> [Driver_1_steer_min_VAL]
  [Driver_1_steer_min_VAL] -> Terminator/1
  [Driver_1_steer_min_TBL] -> Terminator1/1
  Table/1 -> [Driver_1_steer_min_TBL]

== system Demo_veDYNA_cs/Vedyna_Vehicle/CPT_MDL/MDL_PAR/Driver/System Instance 1/steer_rate_max [deg/s] ==
  Table : Lookup  InputValues=CPT.MDL_PAR.Driver{1}.steer_rate_max.Table.x  Table=CPT.MDL_PAR.Driver{1}.steer_rate_max.Table.v  SaturateOnIntegerOverflow=on
  Terminator : Terminator
  Terminator1 : Terminator
  Value : Constant  Value=CPT.MDL_PAR.Driver{1}.steer_rate_max.Value.v
  tag scope: Driver_1_steer_rate_max_TBL=global, Driver_1_steer_rate_max_VAL=global
  wires:
  [vdy_Simctrl_tsim] -> Table/1
  Value/1 -> [Driver_1_steer_rate_max_VAL]
  [Driver_1_steer_rate_max_VAL] -> Terminator/1
  [Driver_1_steer_rate_max_TBL] -> Terminator1/1
  Table/1 -> [Driver_1_steer_rate_max_TBL]

== system Demo_veDYNA_cs/Vedyna_Vehicle/CPT_MDL/MDL_PAR/Driver/System Instance 1/steer_rate_min [deg/s] ==
  Table : Lookup  InputValues=CPT.MDL_PAR.Driver{1}.steer_rate_min.Table.x  Table=CPT.MDL_PAR.Driver{1}.steer_rate_min.Table.v  SaturateOnIntegerOverflow=on
  Terminator : Terminator
  Terminator1 : Terminator
  Value : Constant  Value=CPT.MDL_PAR.Driver{1}.steer_rate_min.Value.v
  tag scope: Driver_1_steer_rate_min_TBL=global, Driver_1_steer_rate_min_VAL=global
  wires:
  [vdy_Simctrl_tsim] -> Table/1
  Value/1 -> [Driver_1_steer_rate_min_VAL]
  [Driver_1_steer_rate_min_VAL] -> Terminator/1
  [Driver_1_steer_rate_min_TBL] -> Terminator1/1
  Table/1 -> [Driver_1_steer_rate_min_TBL]

== system Demo_veDYNA_cs/Vedyna_Vehicle/CPT_MDL/MDL_PAR/Driver/System Instance 1/steer_smooth_t [s] ==
  Table : Lookup  InputValues=CPT.MDL_PAR.Driver{1}.steer_smooth_t.Table.x  Table=CPT.MDL_PAR.Driver{1}.steer_smooth_t.Table.v  SaturateOnIntegerOverflow=on
  Terminator : Terminator
  Terminator1 : Terminator
  Value : Constant  Value=CPT.MDL_PAR.Driver{1}.steer_smooth_t.Value.v
  tag scope: Driver_1_steer_smooth_t_TBL=global, Driver_1_steer_smooth_t_VAL=global
  wires:
  [vdy_Simctrl_tsim] -> Table/1
  Value/1 -> [Driver_1_steer_smooth_t_VAL]
  [Driver_1_steer_smooth_t_VAL] -> Terminator/1
  [Driver_1_steer_smooth_t_TBL] -> Terminator1/1
  Table/1 -> [Driver_1_steer_smooth_t_TBL]

== system Demo_veDYNA_cs/Vedyna_Vehicle/CPT_MDL/MDL_PAR/Driver/System Instance 1/target_aim_x [m] ==
  Table : Lookup  InputValues=CPT.MDL_PAR.Driver{1}.target_aim_x.Table.x  Table=CPT.MDL_PAR.Driver{1}.target_aim_x.Table.v  SaturateOnIntegerOverflow=on
  Terminator : Terminator
  Terminator1 : Terminator
  Value : Constant  Value=CPT.MDL_PAR.Driver{1}.target_aim_x.Value.v
  tag scope: Driver_1_target_aim_x_TBL=global, Driver_1_target_aim_x_VAL=global
  wires:
  [vdy_Simctrl_tsim] -> Table/1
  Value/1 -> [Driver_1_target_aim_x_VAL]
  [Driver_1_target_aim_x_VAL] -> Terminator/1
  [Driver_1_target_aim_x_TBL] -> Terminator1/1
  Table/1 -> [Driver_1_target_aim_x_TBL]

== system Demo_veDYNA_cs/Vedyna_Vehicle/CPT_MDL/MDL_PAR/Driver/System Instance 1/tgt_a_max [m/s^2] ==
  Table : Lookup  InputValues=CPT.MDL_PAR.Driver{1}.tgt_a_max.Table.x  Table=CPT.MDL_PAR.Driver{1}.tgt_a_max.Table.v  SaturateOnIntegerOverflow=on
  Terminator : Terminator
  Terminator1 : Terminator
  Value : Constant  Value=CPT.MDL_PAR.Driver{1}.tgt_a_max.Value.v
  tag scope: Driver_1_tgt_a_max_TBL=global, Driver_1_tgt_a_max_VAL=global
  wires:
  [vdy_Simctrl_tsim] -> Table/1
  Value/1 -> [Driver_1_tgt_a_max_VAL]
  [Driver_1_tgt_a_max_VAL] -> Terminator/1
  [Driver_1_tgt_a_max_TBL] -> Terminator1/1
  Table/1 -> [Driver_1_tgt_a_max_TBL]

== system Demo_veDYNA_cs/Vedyna_Vehicle/CPT_MDL/MDL_PAR/Driver/System Instance 1/tgt_acc_smooth_t [s] ==
  Table : Lookup  InputValues=CPT.MDL_PAR.Driver{1}.tgt_acc_smooth_t.Table.x  Table=CPT.MDL_PAR.Driver{1}.tgt_acc_smooth_t.Table.v  SaturateOnIntegerOverflow=on
  Terminator : Terminator
  Terminator1 : Terminator
  Value : Constant  Value=CPT.MDL_PAR.Driver{1}.tgt_acc_smooth_t.Value.v
  tag scope: Driver_1_tgt_acc_smooth_t_TBL=global, Driver_1_tgt_acc_smooth_t_VAL=global
  wires:
  [vdy_Simctrl_tsim] -> Table/1
  Value/1 -> [Driver_1_tgt_acc_smooth_t_VAL]
  [Driver_1_tgt_acc_smooth_t_VAL] -> Terminator/1
  [Driver_1_tgt_acc_smooth_t_TBL] -> Terminator1/1
  Table/1 -> [Driver_1_tgt_acc_smooth_t_TBL]

== system Demo_veDYNA_cs/Vedyna_Vehicle/CPT_MDL/MDL_PAR/Driver/System Instance 1/tgt_ax_max [m/s^2] ==
  Table : Lookup  InputValues=CPT.MDL_PAR.Driver{1}.tgt_ax_max.Table.x  Table=CPT.MDL_PAR.Driver{1}.tgt_ax_max.Table.v  SaturateOnIntegerOverflow=on
  Terminator : Terminator
  Terminator1 : Terminator
  Value : Constant  Value=CPT.MDL_PAR.Driver{1}.tgt_ax_max.Value.v
  tag scope: Driver_1_tgt_ax_max_TBL=global, Driver_1_tgt_ax_max_VAL=global
  wires:
  [vdy_Simctrl_tsim] -> Table/1
  Value/1 -> [Driver_1_tgt_ax_max_VAL]
  [Driver_1_tgt_ax_max_VAL] -> Terminator/1
  [Driver_1_tgt_ax_max_TBL] -> Terminator1/1
  Table/1 -> [Driver_1_tgt_ax_max_TBL]

== system Demo_veDYNA_cs/Vedyna_Vehicle/CPT_MDL/MDL_PAR/Driver/System Instance 1/tgt_ax_min [m/s^2] ==
  Table : Lookup  InputValues=CPT.MDL_PAR.Driver{1}.tgt_ax_min.Table.x  Table=CPT.MDL_PAR.Driver{1}.tgt_ax_min.Table.v  SaturateOnIntegerOverflow=on
  Terminator : Terminator
  Terminator1 : Terminator
  Value : Constant  Value=CPT.MDL_PAR.Driver{1}.tgt_ax_min.Value.v
  tag scope: Driver_1_tgt_ax_min_TBL=global, Driver_1_tgt_ax_min_VAL=global
  wires:
  [vdy_Simctrl_tsim] -> Table/1
  Value/1 -> [Driver_1_tgt_ax_min_VAL]
  [Driver_1_tgt_ax_min_VAL] -> Terminator/1
  [Driver_1_tgt_ax_min_TBL] -> Terminator1/1
  Table/1 -> [Driver_1_tgt_ax_min_TBL]

== system Demo_veDYNA_cs/Vedyna_Vehicle/CPT_MDL/MDL_PAR/Driver/System Instance 1/tgt_ay_max [m/s^2] ==
  Table : Lookup  InputValues=CPT.MDL_PAR.Driver{1}.tgt_ay_max.Table.x  Table=CPT.MDL_PAR.Driver{1}.tgt_ay_max.Table.v  SaturateOnIntegerOverflow=on
  Terminator : Terminator
  Terminator1 : Terminator
  Value : Constant  Value=CPT.MDL_PAR.Driver{1}.tgt_ay_max.Value.v
  tag scope: Driver_1_tgt_ay_max_TBL=global, Driver_1_tgt_ay_max_VAL=global
  wires:
  [vdy_Simctrl_tsim] -> Table/1
  Value/1 -> [Driver_1_tgt_ay_max_VAL]
  [Driver_1_tgt_ay_max_VAL] -> Terminator/1
  [Driver_1_tgt_ay_max_TBL] -> Terminator1/1
  Table/1 -> [Driver_1_tgt_ay_max_TBL]

== system Demo_veDYNA_cs/Vedyna_Vehicle/CPT_MDL/MDL_PAR/Driver/System Instance 1/tgt_v_max [m/s] ==
  Table : Lookup  InputValues=CPT.MDL_PAR.Driver{1}.tgt_v_max.Table.x  Table=CPT.MDL_PAR.Driver{1}.tgt_v_max.Table.v  SaturateOnIntegerOverflow=on
  Terminator : Terminator
  Terminator1 : Terminator
  Value : Constant  Value=CPT.MDL_PAR.Driver{1}.tgt_v_max.Value.v
  tag scope: Driver_1_tgt_v_max_TBL=global, Driver_1_tgt_v_max_VAL=global
  wires:
  [vdy_Simctrl_tsim] -> Table/1
  Value/1 -> [Driver_1_tgt_v_max_VAL]
  [Driver_1_tgt_v_max_VAL] -> Terminator/1
  [Driver_1_tgt_v_max_TBL] -> Terminator1/1
  Table/1 -> [Driver_1_tgt_v_max_TBL]

== system Demo_veDYNA_cs/Vedyna_Vehicle/CPT_MDL/MDL_PAR/Driver/System Instance 1/tgt_v_min [m/s] ==
  Table : Lookup  InputValues=CPT.MDL_PAR.Driver{1}.tgt_v_min.Table.x  Table=CPT.MDL_PAR.Driver{1}.tgt_v_min.Table.v  SaturateOnIntegerOverflow=on
  Terminator : Terminator
  Terminator1 : Terminator
  Value : Constant  Value=CPT.MDL_PAR.Driver{1}.tgt_v_min.Value.v
  tag scope: Driver_1_tgt_v_min_TBL=global, Driver_1_tgt_v_min_VAL=global
  wires:
  [vdy_Simctrl_tsim] -> Table/1
  Value/1 -> [Driver_1_tgt_v_min_VAL]
  [Driver_1_tgt_v_min_VAL] -> Terminator/1
  [Driver_1_tgt_v_min_TBL] -> Terminator1/1
  Table/1 -> [Driver_1_tgt_v_min_TBL]

== system Demo_veDYNA_cs/Vedyna_Vehicle/CPT_MDL/MDL_PAR/Driver/System Instance 1/use_simulink_sw [-] ==
  Table : Lookup  InputValues=CPT.MDL_PAR.Driver{1}.use_simulink_sw.Table.x  Table=CPT.MDL_PAR.Driver{1}.use_simulink_sw.Table.v  SaturateOnIntegerOverflow=on
  Terminator : Terminator
  Terminator1 : Terminator
  Value : Constant  Value=CPT.MDL_PAR.Driver{1}.use_simulink_sw.Value.v
  tag scope: Driver_1_use_simulink_sw_TBL=global, Driver_1_use_simulink_sw_VAL=global
  wires:
  [vdy_Simctrl_tsim] -> Table/1
  Value/1 -> [Driver_1_use_simulink_sw_VAL]
  [Driver_1_use_simulink_sw_VAL] -> Terminator/1
  [Driver_1_use_simulink_sw_TBL] -> Terminator1/1
  Table/1 -> [Driver_1_use_simulink_sw_TBL]

== system Demo_veDYNA_cs/Vedyna_Vehicle/CPT_MDL/MDL_PAR/Driver/System Instance 1/v_comp_scale [-] ==
  Table : Lookup  InputValues=CPT.MDL_PAR.Driver{1}.v_comp_scale.Table.x  Table=CPT.MDL_PAR.Driver{1}.v_comp_scale.Table.v  SaturateOnIntegerOverflow=on
  Terminator : Terminator
  Terminator1 : Terminator
  Value : Constant  Value=CPT.MDL_PAR.Driver{1}.v_comp_scale.Value.v
  tag scope: Driver_1_v_comp_scale_TBL=global, Driver_1_v_comp_scale_VAL=global
  wires:
  [vdy_Simctrl_tsim] -> Table/1
  Value/1 -> [Driver_1_v_comp_scale_VAL]
  [Driver_1_v_comp_scale_VAL] -> Terminator/1
  [Driver_1_v_comp_scale_TBL] -> Terminator1/1
  Table/1 -> [Driver_1_v_comp_scale_TBL]

== system Demo_veDYNA_cs/Vedyna_Vehicle/CPT_MDL/MDL_PAR/Driver/System Instance 1/v_path [m/s] ==
  Table : Lookup  InputValues=CPT.MDL_PAR.Driver{1}.v_path.Table.x  Table=CPT.MDL_PAR.Driver{1}.v_path.Table.v  SaturateOnIntegerOverflow=on
  Terminator : Terminator
  Terminator1 : Terminator
  Value : Constant  Value=CPT.MDL_PAR.Driver{1}.v_path.Value.v
  tag scope: Driver_1_v_path_TBL=global, Driver_1_v_path_VAL=global
  wires:
  [vdy_Simctrl_tsim] -> Table/1
  Value/1 -> [Driver_1_v_path_VAL]
  [Driver_1_v_path_VAL] -> Terminator/1
  [Driver_1_v_path_TBL] -> Terminator1/1
  Table/1 -> [Driver_1_v_path_TBL]

== system Demo_veDYNA_cs/Vedyna_Vehicle/CPT_MDL/MDL_PAR/Engine/System Instance 1/ASR_Flag [-] ==
  Table : Lookup  InputValues=CPT.MDL_PAR.Engine{1}.ASR_Flag.Table.x  Table=CPT.MDL_PAR.Engine{1}.ASR_Flag.Table.v  SaturateOnIntegerOverflow=on
  Terminator : Terminator
  Terminator1 : Terminator
  Value : Constant  Value=CPT.MDL_PAR.Engine{1}.ASR_Flag.Value.v
  tag scope: Engine_1_ASR_Flag_TBL=global, Engine_1_ASR_Flag_VAL=global
  wires:
  [vdy_Simctrl_tsim] -> Table/1
  Value/1 -> [Engine_1_ASR_Flag_VAL]
  [Engine_1_ASR_Flag_VAL] -> Terminator/1
  [Engine_1_ASR_Flag_TBL] -> Terminator1/1
  Table/1 -> [Engine_1_ASR_Flag_TBL]

== system Demo_veDYNA_cs/Vedyna_Vehicle/CPT_MDL/MDL_PAR/Engine/System Instance 1/ASR_Torque [Nm] ==
  Table : Lookup  InputValues=CPT.MDL_PAR.Engine{1}.ASR_Torque.Table.x  Table=CPT.MDL_PAR.Engine{1}.ASR_Torque.Table.v  SaturateOnIntegerOverflow=on
  Terminator : Terminator
  Terminator1 : Terminator
  Value : Constant  Value=CPT.MDL_PAR.Engine{1}.ASR_Torque.Value.v
  tag scope: Engine_1_ASR_Torque_TBL=global, Engine_1_ASR_Torque_VAL=global
  wires:
  [vdy_Simctrl_tsim] -> Table/1
  Value/1 -> [Engine_1_ASR_Torque_VAL]
  [Engine_1_ASR_Torque_VAL] -> Terminator/1
  [Engine_1_ASR_Torque_TBL] -> Terminator1/1
  Table/1 -> [Engine_1_ASR_Torque_TBL]

== system Demo_veDYNA_cs/Vedyna_Vehicle/CPT_MDL/MDL_PAR/Engine/System Instance 1/MSR_Flag [-] ==
  Table : Lookup  InputValues=CPT.MDL_PAR.Engine{1}.MSR_Flag.Table.x  Table=CPT.MDL_PAR.Engine{1}.MSR_Flag.Table.v  SaturateOnIntegerOverflow=on
  Terminator : Terminator
  Terminator1 : Terminator
  Value : Constant  Value=CPT.MDL_PAR.Engine{1}.MSR_Flag.Value.v
  tag scope: Engine_1_MSR_Flag_TBL=global, Engine_1_MSR_Flag_VAL=global
  wires:
  [vdy_Simctrl_tsim] -> Table/1
  Value/1 -> [Engine_1_MSR_Flag_VAL]
  [Engine_1_MSR_Flag_VAL] -> Terminator/1
  [Engine_1_MSR_Flag_TBL] -> Terminator1/1
  Table/1 -> [Engine_1_MSR_Flag_TBL]

== system Demo_veDYNA_cs/Vedyna_Vehicle/CPT_MDL/MDL_PAR/Engine/System Instance 1/MSR_Torque [Nm] ==
  Table : Lookup  InputValues=CPT.MDL_PAR.Engine{1}.MSR_Torque.Table.x  Table=CPT.MDL_PAR.Engine{1}.MSR_Torque.Table.v  SaturateOnIntegerOverflow=on
  Terminator : Terminator
  Terminator1 : Terminator
  Value : Constant  Value=CPT.MDL_PAR.Engine{1}.MSR_Torque.Value.v
  tag scope: Engine_1_MSR_Torque_TBL=global, Engine_1_MSR_Torque_VAL=global
  wires:
  [vdy_Simctrl_tsim] -> Table/1
  Value/1 -> [Engine_1_MSR_Torque_VAL]
  [Engine_1_MSR_Torque_VAL] -> Terminator/1
  [Engine_1_MSR_Torque_TBL] -> Terminator1/1
  Table/1 -> [Engine_1_MSR_Torque_TBL]

== system Demo_veDYNA_cs/Vedyna_Vehicle/CPT_MDL/MDL_PAR/GearCtrl/System Instance 1/Gear [-] ==
  Table : Lookup  InputValues=CPT.MDL_PAR.GearCtrl{1}.Gear.Table.x  Table=CPT.MDL_PAR.GearCtrl{1}.Gear.Table.v  SaturateOnIntegerOverflow=on
  Terminator : Terminator
  Terminator1 : Terminator
  Value : Constant  Value=CPT.MDL_PAR.GearCtrl{1}.Gear.Value.v
  tag scope: GearCtrl_1_Gear_TBL=global, GearCtrl_1_Gear_VAL=global
  wires:
  [vdy_Simctrl_tsim] -> Table/1
  Value/1 -> [GearCtrl_1_Gear_VAL]
  [GearCtrl_1_Gear_VAL] -> Terminator/1
  [GearCtrl_1_Gear_TBL] -> Terminator1/1
  Table/1 -> [GearCtrl_1_Gear_TBL]

== system Demo_veDYNA_cs/Vedyna_Vehicle/CPT_MDL/MDL_PAR/GearCtrl/System Instance 1/UpShiftRequest [-1,1] ==
  Table : Lookup  InputValues=CPT.MDL_PAR.GearCtrl{1}.UpShiftRequest.Table.x  Table=CPT.MDL_PAR.GearCtrl{1}.UpShiftRequest.Table.v  SaturateOnIntegerOverflow=on
  Terminator : Terminator
  Terminator1 : Terminator
  Value : Constant  Value=CPT.MDL_PAR.GearCtrl{1}.UpShiftRequest.Value.v
  tag scope: GearCtrl_1_UpShiftRequest_TBL=global, GearCtrl_1_UpShiftRequest_VAL=global
  wires:
  [vdy_Simctrl_tsim] -> Table/1
  Value/1 -> [GearCtrl_1_UpShiftRequest_VAL]
  [GearCtrl_1_UpShiftRequest_VAL] -> Terminator/1
  [GearCtrl_1_UpShiftRequest_TBL] -> Terminator1/1
  Table/1 -> [GearCtrl_1_UpShiftRequest_TBL]

== system Demo_veDYNA_cs/Vedyna_Vehicle/CPT_MDL/MDL_PAR/ManLatCtrl/System Instance 1/Curvature [1/m] ==
  Table : Lookup  InputValues=CPT.MDL_PAR.ManLatCtrl{1}.Curvature.Table.x  Table=CPT.MDL_PAR.ManLatCtrl{1}.Curvature.Table.v  SaturateOnIntegerOverflow=on
  Terminator : Terminator
  Terminator1 : Terminator
  Value : Constant  Value=CPT.MDL_PAR.ManLatCtrl{1}.Curvature.Value.v
  tag scope: ManLatCtrl_1_Curvature_TBL=global, ManLatCtrl_1_Curvature_VAL=global
  wires:
  [vdy_Simctrl_tsim] -> Table/1
  Value/1 -> [ManLatCtrl_1_Curvature_VAL]
  [ManLatCtrl_1_Curvature_VAL] -> Terminator/1
  [ManLatCtrl_1_Curvature_TBL] -> Terminator1/1
  Table/1 -> [ManLatCtrl_1_Curvature_TBL]

== system Demo_veDYNA_cs/Vedyna_Vehicle/CPT_MDL/MDL_PAR/ManLatCtrl/System Instance 1/Steering [deg] ==
  Table : Lookup  InputValues=CPT.MDL_PAR.ManLatCtrl{1}.Steering.Table.x  Table=CPT.MDL_PAR.ManLatCtrl{1}.Steering.Table.v  SaturateOnIntegerOverflow=on
  Terminator : Terminator
  Terminator1 : Terminator
  Value : Constant  Value=CPT.MDL_PAR.ManLatCtrl{1}.Steering.Value.v
  tag scope: ManLatCtrl_1_Steering_TBL=global, ManLatCtrl_1_Steering_VAL=global
  wires:
  [vdy_Simctrl_tsim] -> Table/1
  Value/1 -> [ManLatCtrl_1_Steering_VAL]
  [ManLatCtrl_1_Steering_VAL] -> Terminator/1
  [ManLatCtrl_1_Steering_TBL] -> Terminator1/1
  Table/1 -> [ManLatCtrl_1_Steering_TBL]
